simulink model "pid_hiv_forskjellige"  (R2023b)
settings: Solver=VariableStepAuto  StartTime=0.0  StopTime=15  RelTol=1e-6
undefined symbols (not defined in the file): areal_topp, Cd_topp, g, masse, tetthet_vann
libraries: spsFirstOrderFilterLib x4
settings Model: Creator=kristianbirkeland  LastModifiedBy=bmm1
settings DebuggingCC: UnconnectedInputMsg=warning  UnconnectedOutputMsg=warning  UnconnectedLineMsg=warning
settings ModelReferenceCC: EnableRefExpFcnMdlSchedulingChecks=on
settings RTWCC: DLArmComputeVersion=19.05

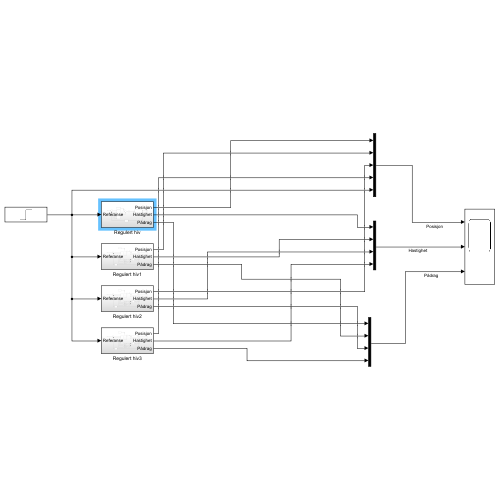
[thumbnail: Simulink's stored preview of the top-level diagram]
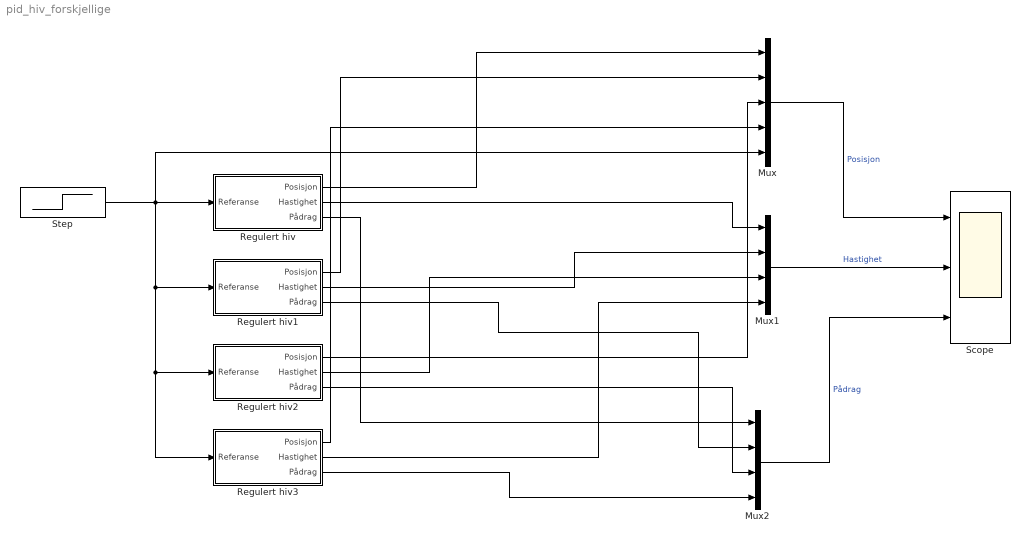
== system pid_hiv_forskjellige ==
  Mux : Mux  Inputs=5
  Mux1 : Mux
  Mux2 : Mux
  Regulert hiv : Subsystem
  Regulert hiv1 : Subsystem
  Regulert hiv2 : Subsystem
  Regulert hiv3 : Subsystem
  Scope : Scope  NumInputPorts=3
  Step : Step  After=0.6  SampleTime=0
  wires:
  Step/1 -> Regulert hiv3/1(Referanse), Regulert hiv2/1(Referanse), Regulert hiv1/1(Referanse), Mux/5, Regulert hiv/1(Referanse)
  Mux/1 -> Scope/1  "Posisjon"
  Regulert hiv/1(Posisjon) -> Mux/1
  Regulert hiv1/1(Posisjon) -> Mux/2
  Regulert hiv2/1(Posisjon) -> Mux/3
  Regulert hiv3/1(Posisjon) -> Mux/4
  Regulert hiv/2(Hastighet) -> Mux1/1
  Regulert hiv1/2(Hastighet) -> Mux1/2
  Regulert hiv2/2(Hastighet) -> Mux1/3
  Regulert hiv3/2(Hastighet) -> Mux1/4
  Regulert hiv3/3(Pådrag) -> Mux2/4
  Regulert hiv2/3(Pådrag) -> Mux2/3
  Regulert hiv1/3(Pådrag) -> Mux2/2
  Regulert hiv/3(Pådrag) -> Mux2/1
  Mux1/1 -> Scope/2  "Hastighet"
  Mux2/1 -> Scope/3  "Pådrag"

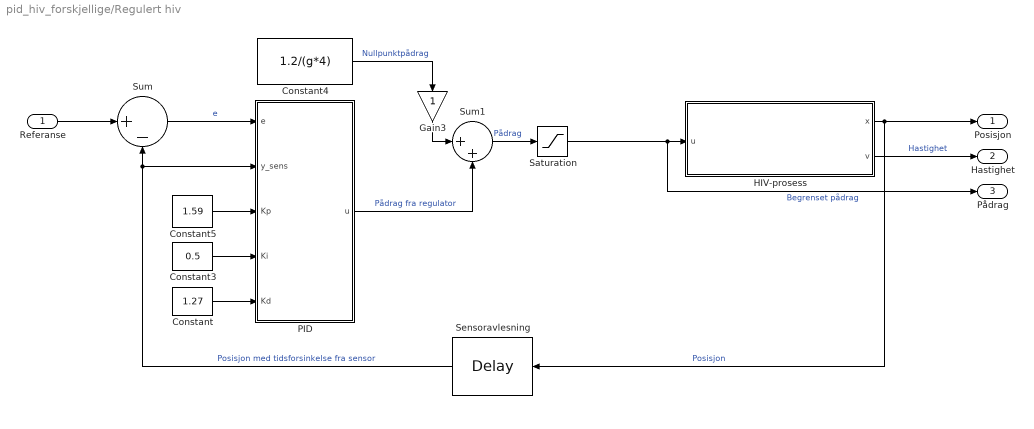
== system pid_hiv_forskjellige/Regulert hiv ==
  Referanse : Inport
  Constant : Constant  Value=1.27
  Constant3 : Constant  Value=0.5
  Constant4 : Constant  Value=1.2/(g*4)
  Constant5 : Constant  Value=1.59
  Gain3 : Gain
  HIV-prosess : Subsystem
      settings: AttributesFormatString=Hiv-modell
  PID : Subsystem
  Saturation : Saturate  UpperLimit=2.7  LowerLimit=-2.7
  Sensoravlesning : TransportDelay  DelayTime=0.2
  Sum : Sum  Inputs=|+-
  Sum1 : Sum  Inputs=|++
  Posisjon : Outport
  Hastighet : Outport  Port=2
  Pådrag : Outport  Port=3
  wires:
  PID/1(u) -> Sum1/2  "Pådrag fra regulator"
  Sum/1 -> PID/1(e)  "e"
  Constant/1 -> PID/5(Kd)
  Gain3/1 -> Sum1/1
  Sensoravlesning/1 -> Sum/2, PID/2(y_sens)  "Posisjon med tidsforsinkelse fra sensor"
  HIV-prosess/1(x) -> Posisjon/1, Sensoravlesning/1  "Posisjon"
  HIV-prosess/2(v) -> Hastighet/1  "Hastighet"
  Referanse/1 -> Sum/1
  Sum1/1 -> Saturation/1  "Pådrag"
  Constant4/1 -> Gain3/1  "Nullpunktpådrag"
  Saturation/1 -> HIV-prosess/1(u), Pådrag/1  "Begrenset pådrag"
  Constant3/1 -> PID/4(Ki)
  Constant5/1 -> PID/3(Kp)

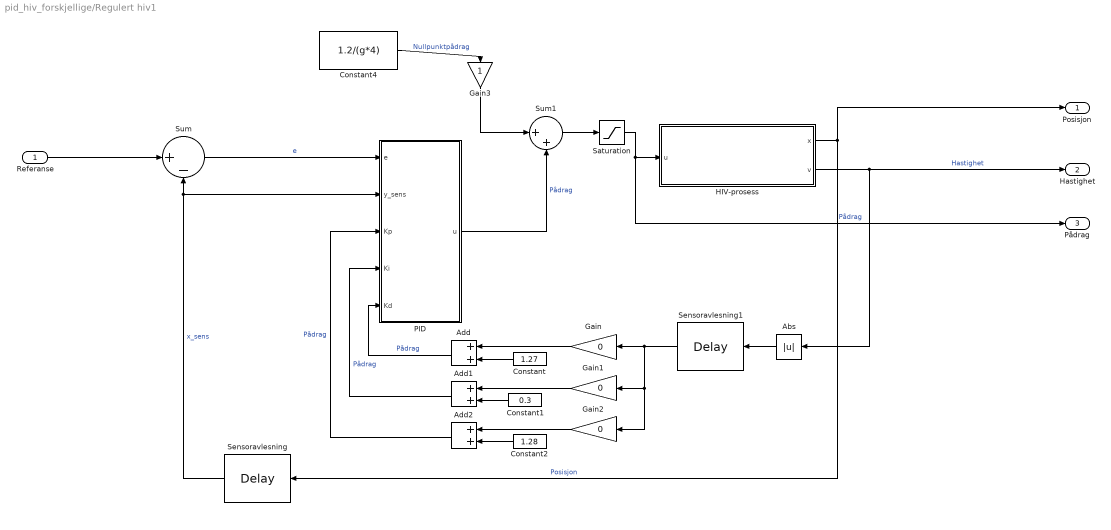
== system pid_hiv_forskjellige/Regulert hiv1 ==
  Referanse : Inport
  Abs : Abs  SaturateOnIntegerOverflow=off
  Add : Sum
  Add1 : Sum
  Add2 : Sum
  Constant : Constant  Value=1.27
  Constant1 : Constant  Value=0.3
  Constant2 : Constant  Value=1.28
  Constant4 : Constant  Value=1.2/(g*4)
  Gain : Gain  Gain=0
  Gain1 : Gain  Gain=0
  Gain2 : Gain  Gain=0
  Gain3 : Gain
  HIV-prosess : Subsystem
      settings: AttributesFormatString=Hiv-modell
  PID : Subsystem
  Saturation : Saturate  UpperLimit=2.7  LowerLimit=-2.7
  Sensoravlesning : TransportDelay  DelayTime=0.2
  Sensoravlesning1 : TransportDelay  DelayTime=0.15
  Sum : Sum  Inputs=|+-
  Sum1 : Sum  Inputs=|++
  Posisjon : Outport
  Hastighet : Outport  Port=2
  Pådrag : Outport  Port=3
  wires:
  PID/1(u) -> Sum1/2  "Pådrag"
  Gain2/1 -> Add2/1
  Add/1 -> PID/5(Kd)  "Pådrag"
  Gain1/1 -> Add1/1
  Sum/1 -> PID/1(e)  "e"
  Constant2/1 -> Add2/2
  Gain/1 -> Add/1
  Abs/1 -> Sensoravlesning1/1
  Add1/1 -> PID/4(Ki)  "Pådrag"
  Constant/1 -> Add/2
  Add2/1 -> PID/3(Kp)  "Pådrag"
  Sensoravlesning1/1 -> Gain2/1, Gain1/1, Gain/1
  Constant1/1 -> Add1/2
  Gain3/1 -> Sum1/1
  Sensoravlesning/1 -> Sum/2, PID/2(y_sens)  "x_sens"
  HIV-prosess/1(x) -> Posisjon/1, Sensoravlesning/1  "Posisjon"
  HIV-prosess/2(v) -> Hastighet/1, Abs/1  "Hastighet"
  Referanse/1 -> Sum/1
  Sum1/1 -> Saturation/1
  Constant4/1 -> Gain3/1  "Nullpunktpådrag"
  Saturation/1 -> Pådrag/1, HIV-prosess/1(u)  "Pådrag"

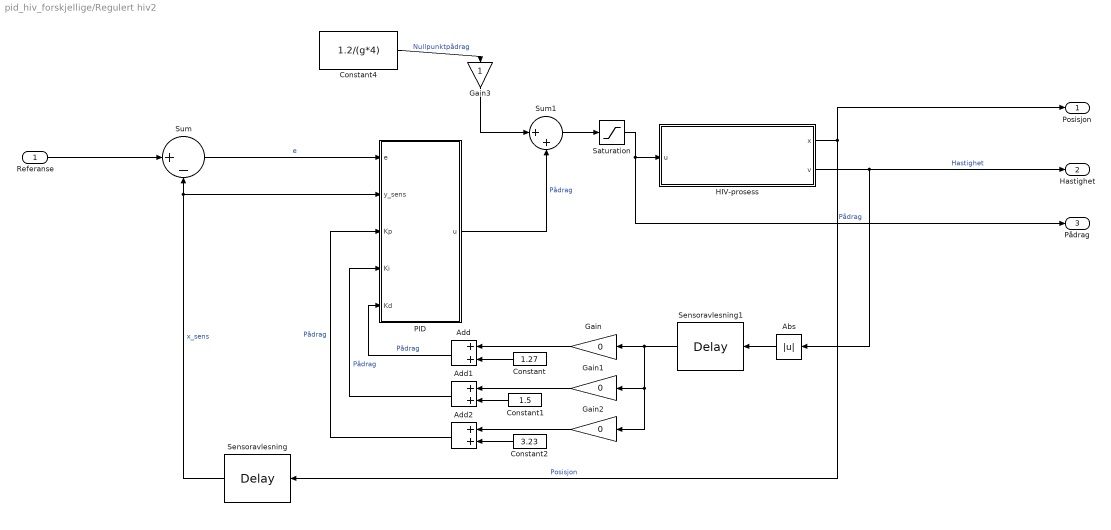
== system pid_hiv_forskjellige/Regulert hiv2 ==
  Referanse : Inport
  Abs : Abs  SaturateOnIntegerOverflow=off
  Add : Sum
  Add1 : Sum
  Add2 : Sum
  Constant : Constant  Value=1.27
  Constant1 : Constant  Value=1.5
  Constant2 : Constant  Value=3.23
  Constant4 : Constant  Value=1.2/(g*4)
  Gain : Gain  Gain=0
  Gain1 : Gain  Gain=0
  Gain2 : Gain  Gain=0
  Gain3 : Gain
  HIV-prosess : Subsystem
      settings: AttributesFormatString=Hiv-modell
  PID : Subsystem
  Saturation : Saturate  UpperLimit=2.7  LowerLimit=-2.7
  Sensoravlesning : TransportDelay  DelayTime=0.2
  Sensoravlesning1 : TransportDelay  DelayTime=0.15
  Sum : Sum  Inputs=|+-
  Sum1 : Sum  Inputs=|++
  Posisjon : Outport
  Hastighet : Outport  Port=2
  Pådrag : Outport  Port=3
  wires:
  PID/1(u) -> Sum1/2  "Pådrag"
  Gain2/1 -> Add2/1
  Add/1 -> PID/5(Kd)  "Pådrag"
  Gain1/1 -> Add1/1
  Sum/1 -> PID/1(e)  "e"
  Constant2/1 -> Add2/2
  Gain/1 -> Add/1
  Abs/1 -> Sensoravlesning1/1
  Add1/1 -> PID/4(Ki)  "Pådrag"
  Constant/1 -> Add/2
  Add2/1 -> PID/3(Kp)  "Pådrag"
  Sensoravlesning1/1 -> Gain2/1, Gain1/1, Gain/1
  Constant1/1 -> Add1/2
  Gain3/1 -> Sum1/1
  Sensoravlesning/1 -> Sum/2, PID/2(y_sens)  "x_sens"
  HIV-prosess/1(x) -> Posisjon/1, Sensoravlesning/1  "Posisjon"
  HIV-prosess/2(v) -> Hastighet/1, Abs/1  "Hastighet"
  Referanse/1 -> Sum/1
  Sum1/1 -> Saturation/1
  Constant4/1 -> Gain3/1  "Nullpunktpådrag"
  Saturation/1 -> Pådrag/1, HIV-prosess/1(u)  "Pådrag"

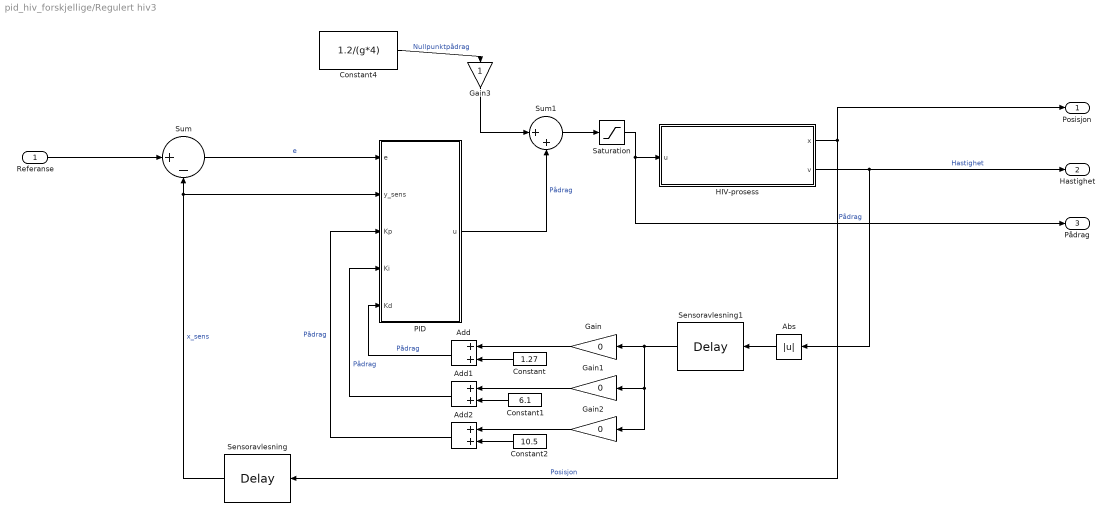
== system pid_hiv_forskjellige/Regulert hiv3 ==
  Referanse : Inport
  Abs : Abs  SaturateOnIntegerOverflow=off
  Add : Sum
  Add1 : Sum
  Add2 : Sum
  Constant : Constant  Value=1.27
  Constant1 : Constant  Value=6.1
  Constant2 : Constant  Value=10.5
  Constant4 : Constant  Value=1.2/(g*4)
  Gain : Gain  Gain=0
  Gain1 : Gain  Gain=0
  Gain2 : Gain  Gain=0
  Gain3 : Gain
  HIV-prosess : Subsystem
      settings: AttributesFormatString=Hiv-modell
  PID : Subsystem
  Saturation : Saturate  UpperLimit=2.7  LowerLimit=-2.7
  Sensoravlesning : TransportDelay  DelayTime=0.2
  Sensoravlesning1 : TransportDelay  DelayTime=0.15
  Sum : Sum  Inputs=|+-
  Sum1 : Sum  Inputs=|++
  Posisjon : Outport
  Hastighet : Outport  Port=2
  Pådrag : Outport  Port=3
  wires:
  PID/1(u) -> Sum1/2  "Pådrag"
  Gain2/1 -> Add2/1
  Add/1 -> PID/5(Kd)  "Pådrag"
  Gain1/1 -> Add1/1
  Sum/1 -> PID/1(e)  "e"
  Constant2/1 -> Add2/2
  Gain/1 -> Add/1
  Abs/1 -> Sensoravlesning1/1
  Add1/1 -> PID/4(Ki)  "Pådrag"
  Constant/1 -> Add/2
  Add2/1 -> PID/3(Kp)  "Pådrag"
  Sensoravlesning1/1 -> Gain2/1, Gain1/1, Gain/1
  Constant1/1 -> Add1/2
  Gain3/1 -> Sum1/1
  Sensoravlesning/1 -> Sum/2, PID/2(y_sens)  "x_sens"
  HIV-prosess/1(x) -> Posisjon/1, Sensoravlesning/1  "Posisjon"
  HIV-prosess/2(v) -> Hastighet/1, Abs/1  "Hastighet"
  Referanse/1 -> Sum/1
  Sum1/1 -> Saturation/1
  Constant4/1 -> Gain3/1  "Nullpunktpådrag"
  Saturation/1 -> Pådrag/1, HIV-prosess/1(u)  "Pådrag"

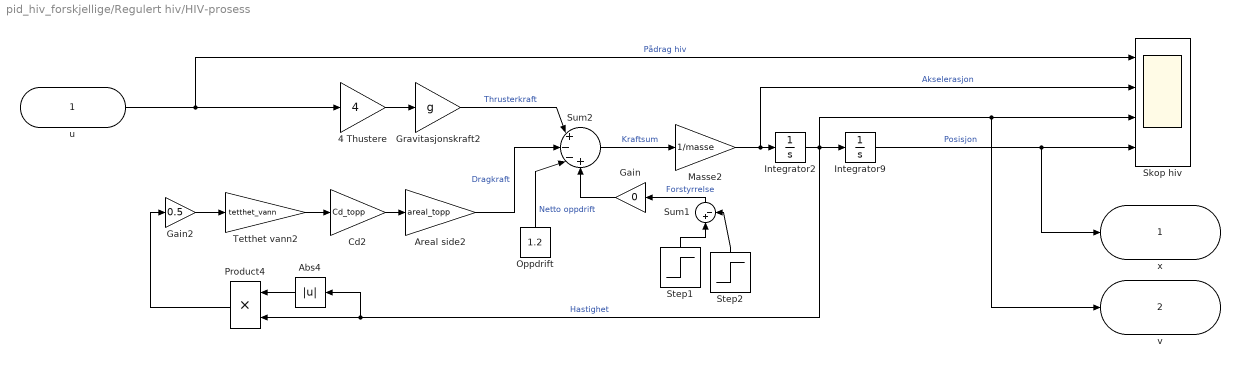
== system pid_hiv_forskjellige/Regulert hiv/HIV-prosess ==
  u : Inport
  4 Thustere : Gain  Gain=4
  Abs4 : Abs  SaturateOnIntegerOverflow=off
  Areal side2 : Gain  Gain=areal_topp
  Cd2 : Gain  Gain=Cd_topp
  Gain : Gain  Gain=0
  Gain2 : Gain  Gain=0.5
  Gravitasjonskraft2 : Gain  Gain=g
  Integrator2 : Integrator
  Integrator9 : Integrator
  Masse2 : Gain  Gain=1/masse
  Oppdrift : Constant  Value=1.2
  Product4 : Product
  Skop hiv : Scope  NumInputPorts=4
  Step1 : Step  Time=10  After=10  SampleTime=0
  Step2 : Step  Time=25  After=10  SampleTime=0
  Sum1 : Sum  Inputs=|+-
  Sum2 : Sum  Inputs=|+--+
  Tetthet vann2 : Gain  Gain=tetthet_vann
  x : Outport
  v : Outport  Port=2
  wires:
  Abs4/1 -> Product4/1
  4 Thustere/1 -> Gravitasjonskraft2/1
  Cd2/1 -> Areal side2/1
  Tetthet vann2/1 -> Cd2/1
  Sum2/1 -> Masse2/1  "Kraftsum"
  Areal side2/1 -> Sum2/2  "Dragkraft"
  Masse2/1 -> Skop hiv/2, Integrator2/1  "Akselerasjon"
  Gain2/1 -> Tetthet vann2/1
  Gravitasjonskraft2/1 -> Sum2/1  "Thrusterkraft"
  Oppdrift/1 -> Sum2/3  "Netto oppdrift"
  Integrator2/1 -> Abs4/1, Product4/2, Integrator9/1, v/1, Skop hiv/3  "Hastighet"
  Product4/1 -> Gain2/1
  u/1 -> Skop hiv/1, 4 Thustere/1  "Pådrag hiv"
  Integrator9/1 -> x/1, Skop hiv/4  "Posisjon"
  Step2/1 -> Sum1/2
  Sum1/1 -> Gain/1  "Forstyrrelse"
  Step1/1 -> Sum1/1
  Gain/1 -> Sum2/4

== system pid_hiv_forskjellige/Regulert hiv/PID ==
  e : Inport
  y_sens : Inport  Port=2
  Kp : Inport  Port=3
  Ki : Inport  Port=4
  Kd : Inport  Port=5
  Derivative : Derivative
  Gain : Gain  Gain=-1
  Integrator : Integrator  LimitOutput=on  UpperSaturationLimit=2  LowerSaturationLimit=-0.15
  Lavpassfilter : spsFirstOrderFilterLib/First-Order Filter  FilterType=Lowpass  Tc=(1.27/1.59)*0.05  Ts=0  Initialize=on  Vac_Init=[0, 0, 60]  Vdc_Init=0  PlotResponse=off  FreqRange="[0,  200,  1]"
  Product : Product
  Product1 : Product
  Product2 : Product
  Scope : Scope  NumInputPorts=3
  Sum : Sum  Inputs=|+++
  u : Outport
  wires:
  e/1 -> Product/2, Product2/1
  Sum/1 -> u/1
  y_sens/1 -> Gain/1
  Lavpassfilter/1 -> Product1/1
  Kd/1 -> Product1/2
  Ki/1 -> Product2/2
  Product2/1 -> Integrator/1
  Product1/1 -> Derivative/1
  Derivative/1 -> Sum/3, Scope/3  "D-Ledd"
  Gain/1 -> Lavpassfilter/1
  Product/1 -> Scope/1, Sum/1  "P-Ledd"
  Integrator/1 -> Sum/2, Scope/2  "I_Ledd"
  Kp/1 -> Product/1

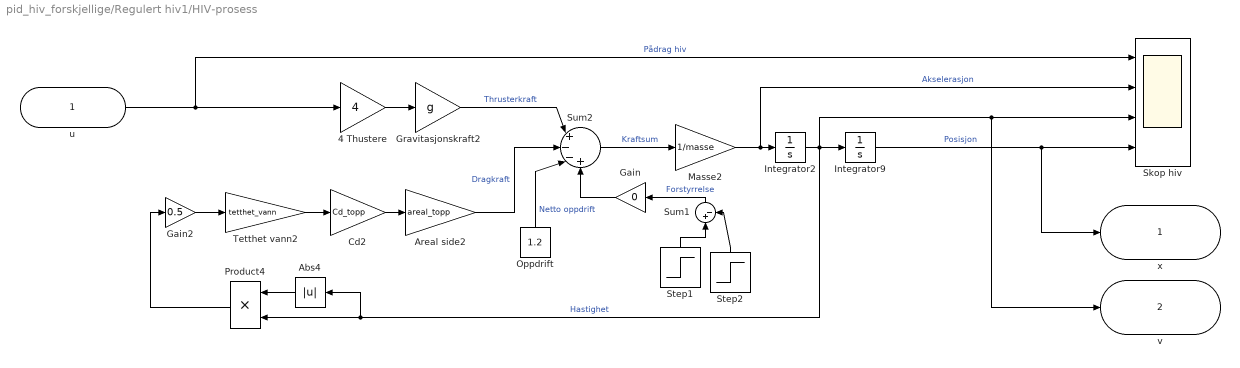
== system pid_hiv_forskjellige/Regulert hiv1/HIV-prosess ==
  u : Inport
  4 Thustere : Gain  Gain=4
  Abs4 : Abs  SaturateOnIntegerOverflow=off
  Areal side2 : Gain  Gain=areal_topp
  Cd2 : Gain  Gain=Cd_topp
  Gain : Gain  Gain=0
  Gain2 : Gain  Gain=0.5
  Gravitasjonskraft2 : Gain  Gain=g
  Integrator2 : Integrator
  Integrator9 : Integrator
  Masse2 : Gain  Gain=1/masse
  Oppdrift : Constant  Value=1.2
  Product4 : Product
  Skop hiv : Scope  NumInputPorts=4
  Step1 : Step  Time=10  After=10  SampleTime=0
  Step2 : Step  Time=25  After=10  SampleTime=0
  Sum1 : Sum  Inputs=|+-
  Sum2 : Sum  Inputs=|+--+
  Tetthet vann2 : Gain  Gain=tetthet_vann
  x : Outport
  v : Outport  Port=2
  wires:
  Abs4/1 -> Product4/1
  4 Thustere/1 -> Gravitasjonskraft2/1
  Cd2/1 -> Areal side2/1
  Tetthet vann2/1 -> Cd2/1
  Sum2/1 -> Masse2/1  "Kraftsum"
  Areal side2/1 -> Sum2/2  "Dragkraft"
  Masse2/1 -> Skop hiv/2, Integrator2/1  "Akselerasjon"
  Gain2/1 -> Tetthet vann2/1
  Gravitasjonskraft2/1 -> Sum2/1  "Thrusterkraft"
  Oppdrift/1 -> Sum2/3  "Netto oppdrift"
  Integrator2/1 -> Abs4/1, Product4/2, Integrator9/1, v/1, Skop hiv/3  "Hastighet"
  Product4/1 -> Gain2/1
  u/1 -> Skop hiv/1, 4 Thustere/1  "Pådrag hiv"
  Integrator9/1 -> x/1, Skop hiv/4  "Posisjon"
  Step2/1 -> Sum1/2
  Sum1/1 -> Gain/1  "Forstyrrelse"
  Step1/1 -> Sum1/1
  Gain/1 -> Sum2/4

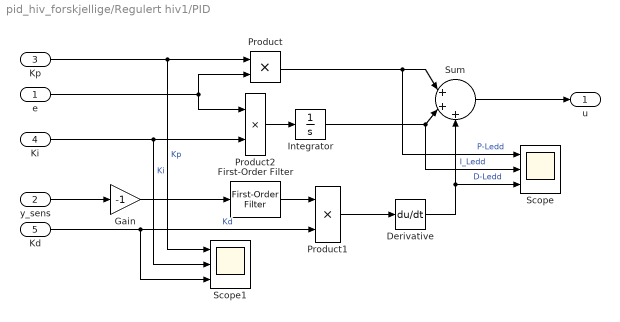
== system pid_hiv_forskjellige/Regulert hiv1/PID ==
  e : Inport
  y_sens : Inport  Port=2
  Kp : Inport  Port=3
  Ki : Inport  Port=4
  Kd : Inport  Port=5
  Derivative : Derivative
  First-Order Filter : spsFirstOrderFilterLib/First-Order Filter  FilterType=Lowpass  Tc=(1.27/1.28)*0.05  Ts=0  Initialize=on  Vac_Init=[0, 0, 60]  Vdc_Init=0  PlotResponse=off  FreqRange="[0,  200,  1]"
  Gain : Gain  Gain=-1
  Integrator : Integrator  LimitOutput=on  UpperSaturationLimit=2  LowerSaturationLimit=-0.15
  Product : Product
  Product1 : Product
  Product2 : Product
  Scope : Scope  NumInputPorts=3
  Scope1 : Scope  NumInputPorts=3
  Sum : Sum  Inputs=|+++
  u : Outport
  wires:
  e/1 -> Product2/1, Product/2
  Sum/1 -> u/1
  y_sens/1 -> Gain/1
  First-Order Filter/1 -> Product1/1
  Kd/1 -> Scope1/3, Product1/2  "Kd"
  Ki/1 -> Scope1/2, Product2/2  "Ki"
  Product2/1 -> Integrator/1
  Product1/1 -> Derivative/1
  Derivative/1 -> Sum/3, Scope/3  "D-Ledd"
  Gain/1 -> First-Order Filter/1
  Product/1 -> Scope/1, Sum/1  "P-Ledd"
  Integrator/1 -> Sum/2, Scope/2  "I_Ledd"
  Kp/1 -> Scope1/1, Product/1  "Kp"

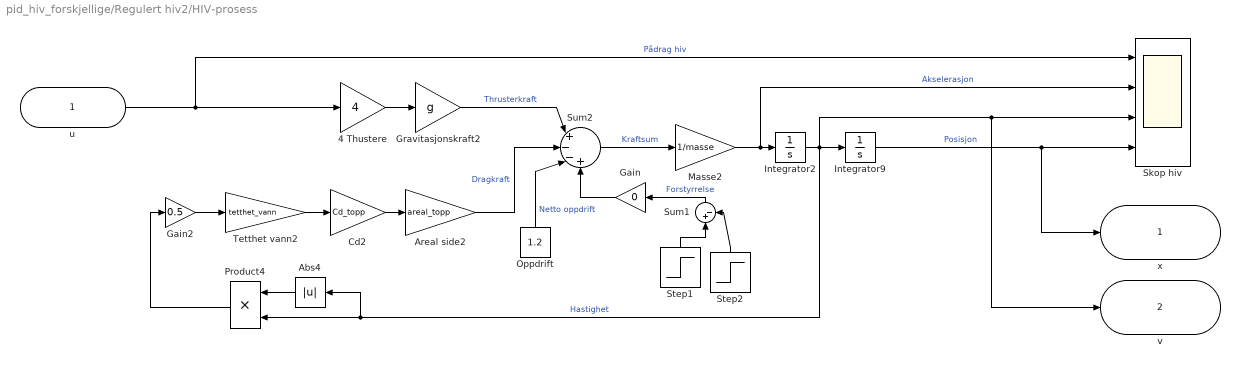
== system pid_hiv_forskjellige/Regulert hiv2/HIV-prosess ==
  u : Inport
  4 Thustere : Gain  Gain=4
  Abs4 : Abs  SaturateOnIntegerOverflow=off
  Areal side2 : Gain  Gain=areal_topp
  Cd2 : Gain  Gain=Cd_topp
  Gain : Gain  Gain=0
  Gain2 : Gain  Gain=0.5
  Gravitasjonskraft2 : Gain  Gain=g
  Integrator2 : Integrator
  Integrator9 : Integrator
  Masse2 : Gain  Gain=1/masse
  Oppdrift : Constant  Value=1.2
  Product4 : Product
  Skop hiv : Scope  NumInputPorts=4
  Step1 : Step  Time=10  After=10  SampleTime=0
  Step2 : Step  Time=25  After=10  SampleTime=0
  Sum1 : Sum  Inputs=|+-
  Sum2 : Sum  Inputs=|+--+
  Tetthet vann2 : Gain  Gain=tetthet_vann
  x : Outport
  v : Outport  Port=2
  wires:
  Abs4/1 -> Product4/1
  4 Thustere/1 -> Gravitasjonskraft2/1
  Cd2/1 -> Areal side2/1
  Tetthet vann2/1 -> Cd2/1
  Sum2/1 -> Masse2/1  "Kraftsum"
  Areal side2/1 -> Sum2/2  "Dragkraft"
  Masse2/1 -> Skop hiv/2, Integrator2/1  "Akselerasjon"
  Gain2/1 -> Tetthet vann2/1
  Gravitasjonskraft2/1 -> Sum2/1  "Thrusterkraft"
  Oppdrift/1 -> Sum2/3  "Netto oppdrift"
  Integrator2/1 -> Abs4/1, Product4/2, Integrator9/1, v/1, Skop hiv/3  "Hastighet"
  Product4/1 -> Gain2/1
  u/1 -> Skop hiv/1, 4 Thustere/1  "Pådrag hiv"
  Integrator9/1 -> x/1, Skop hiv/4  "Posisjon"
  Step2/1 -> Sum1/2
  Sum1/1 -> Gain/1  "Forstyrrelse"
  Step1/1 -> Sum1/1
  Gain/1 -> Sum2/4

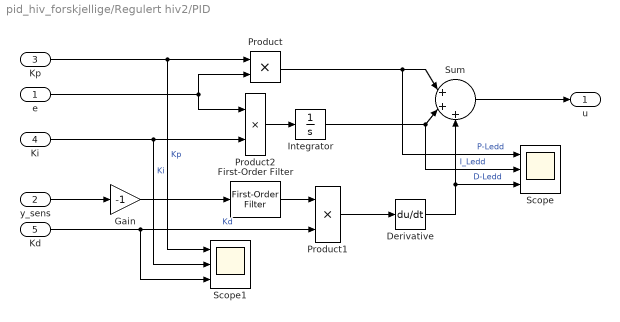
== system pid_hiv_forskjellige/Regulert hiv2/PID ==
  e : Inport
  y_sens : Inport  Port=2
  Kp : Inport  Port=3
  Ki : Inport  Port=4
  Kd : Inport  Port=5
  Derivative : Derivative
  First-Order Filter : spsFirstOrderFilterLib/First-Order Filter  FilterType=Lowpass  Tc=(1.27/3.23)*0.05  Ts=0  Initialize=on  Vac_Init=[0, 0, 60]  Vdc_Init=0  PlotResponse=off  FreqRange="[0,  200,  1]"
  Gain : Gain  Gain=-1
  Integrator : Integrator  LimitOutput=on  UpperSaturationLimit=2  LowerSaturationLimit=-0.15
  Product : Product
  Product1 : Product
  Product2 : Product
  Scope : Scope  NumInputPorts=3
  Scope1 : Scope  NumInputPorts=3
  Sum : Sum  Inputs=|+++
  u : Outport
  wires:
  e/1 -> Product2/1, Product/2
  Sum/1 -> u/1
  y_sens/1 -> Gain/1
  First-Order Filter/1 -> Product1/1
  Kd/1 -> Scope1/3, Product1/2  "Kd"
  Ki/1 -> Scope1/2, Product2/2  "Ki"
  Product2/1 -> Integrator/1
  Product1/1 -> Derivative/1
  Derivative/1 -> Sum/3, Scope/3  "D-Ledd"
  Gain/1 -> First-Order Filter/1
  Product/1 -> Scope/1, Sum/1  "P-Ledd"
  Integrator/1 -> Sum/2, Scope/2  "I_Ledd"
  Kp/1 -> Scope1/1, Product/1  "Kp"

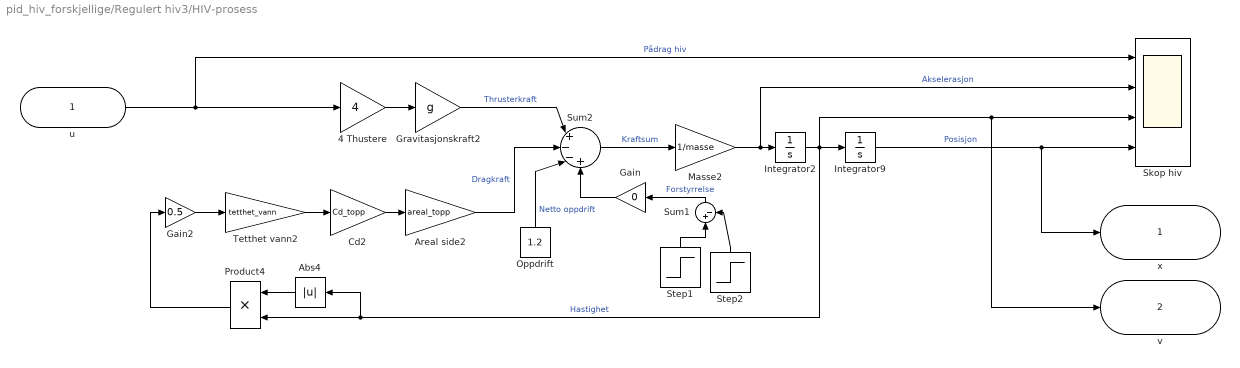
== system pid_hiv_forskjellige/Regulert hiv3/HIV-prosess ==
  u : Inport
  4 Thustere : Gain  Gain=4
  Abs4 : Abs  SaturateOnIntegerOverflow=off
  Areal side2 : Gain  Gain=areal_topp
  Cd2 : Gain  Gain=Cd_topp
  Gain : Gain  Gain=0
  Gain2 : Gain  Gain=0.5
  Gravitasjonskraft2 : Gain  Gain=g
  Integrator2 : Integrator
  Integrator9 : Integrator
  Masse2 : Gain  Gain=1/masse
  Oppdrift : Constant  Value=1.2
  Product4 : Product
  Skop hiv : Scope  NumInputPorts=4
  Step1 : Step  Time=10  After=10  SampleTime=0
  Step2 : Step  Time=25  After=10  SampleTime=0
  Sum1 : Sum  Inputs=|+-
  Sum2 : Sum  Inputs=|+--+
  Tetthet vann2 : Gain  Gain=tetthet_vann
  x : Outport
  v : Outport  Port=2
  wires:
  Abs4/1 -> Product4/1
  4 Thustere/1 -> Gravitasjonskraft2/1
  Cd2/1 -> Areal side2/1
  Tetthet vann2/1 -> Cd2/1
  Sum2/1 -> Masse2/1  "Kraftsum"
  Areal side2/1 -> Sum2/2  "Dragkraft"
  Masse2/1 -> Skop hiv/2, Integrator2/1  "Akselerasjon"
  Gain2/1 -> Tetthet vann2/1
  Gravitasjonskraft2/1 -> Sum2/1  "Thrusterkraft"
  Oppdrift/1 -> Sum2/3  "Netto oppdrift"
  Integrator2/1 -> Abs4/1, Product4/2, Integrator9/1, v/1, Skop hiv/3  "Hastighet"
  Product4/1 -> Gain2/1
  u/1 -> Skop hiv/1, 4 Thustere/1  "Pådrag hiv"
  Integrator9/1 -> x/1, Skop hiv/4  "Posisjon"
  Step2/1 -> Sum1/2
  Sum1/1 -> Gain/1  "Forstyrrelse"
  Step1/1 -> Sum1/1
  Gain/1 -> Sum2/4

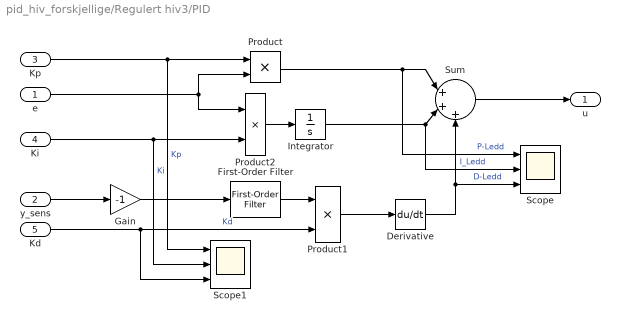
== system pid_hiv_forskjellige/Regulert hiv3/PID ==
  e : Inport
  y_sens : Inport  Port=2
  Kp : Inport  Port=3
  Ki : Inport  Port=4
  Kd : Inport  Port=5
  Derivative : Derivative
  First-Order Filter : spsFirstOrderFilterLib/First-Order Filter  FilterType=Lowpass  Tc=(1.27/10.55)*0.05  Ts=0  Initialize=on  Vac_Init=[0, 0, 60]  Vdc_Init=0  PlotResponse=off  FreqRange="[0,  200,  1]"
  Gain : Gain  Gain=-1
  Integrator : Integrator  LimitOutput=on  UpperSaturationLimit=2  LowerSaturationLimit=-0.15
  Product : Product
  Product1 : Product
  Product2 : Product
  Scope : Scope  NumInputPorts=3
  Scope1 : Scope  NumInputPorts=3
  Sum : Sum  Inputs=|+++
  u : Outport
  wires:
  e/1 -> Product2/1, Product/2
  Sum/1 -> u/1
  y_sens/1 -> Gain/1
  First-Order Filter/1 -> Product1/1
  Kd/1 -> Scope1/3, Product1/2  "Kd"
  Ki/1 -> Scope1/2, Product2/2  "Ki"
  Product2/1 -> Integrator/1
  Product1/1 -> Derivative/1
  Derivative/1 -> Sum/3, Scope/3  "D-Ledd"
  Gain/1 -> First-Order Filter/1
  Product/1 -> Scope/1, Sum/1  "P-Ledd"
  Integrator/1 -> Sum/2, Scope/2  "I_Ledd"
  Kp/1 -> Scope1/1, Product/1  "Kp"
